simulink model "my_PMSM"  (Simulink 8.6)
settings: Solver=ode45  StartTime=0.0  StopTime=2  MaxStep=1e-5  RelTol=1e-3
model workspace (MAT data in the model file):
  Ld = 0.00019
  Lq = 0.00051
  PP = 4
  fluxM = 0.0814
values from neighbouring files (symbols this model uses):
  fluxM = 0.0814    [aaa.mat]
  Ld = 0.00019    [aaa.mat]    (also in param.m = 2e-05)
  Lq = 0.00051    [aaa.mat]    (also in param.m = 4e-05)
  PP = 4    [aaa.mat]
undefined symbols (not defined in the file or in its folder): Vdc
libraries: powerlib x6, powerlib_extras x4, simulink x1
settings Model: Creator=lenovo  LastModifiedBy=Administrator
settings OptimizationCC: InitFltsAndDblsToZero=on
settings DebuggingCC: SaveWithParameterizedLinksMsg=none  SignalResolutionControl=TryResolveAllWithWarning  MultiTaskDSMMsg=warning  MultiTaskCondExecSysMsg=none  FcnCallInpInsideContextMsg=UseLocalSettings
settings GRTTargetCC: TargetFcnLib=ansi_tfl_tmw.mat

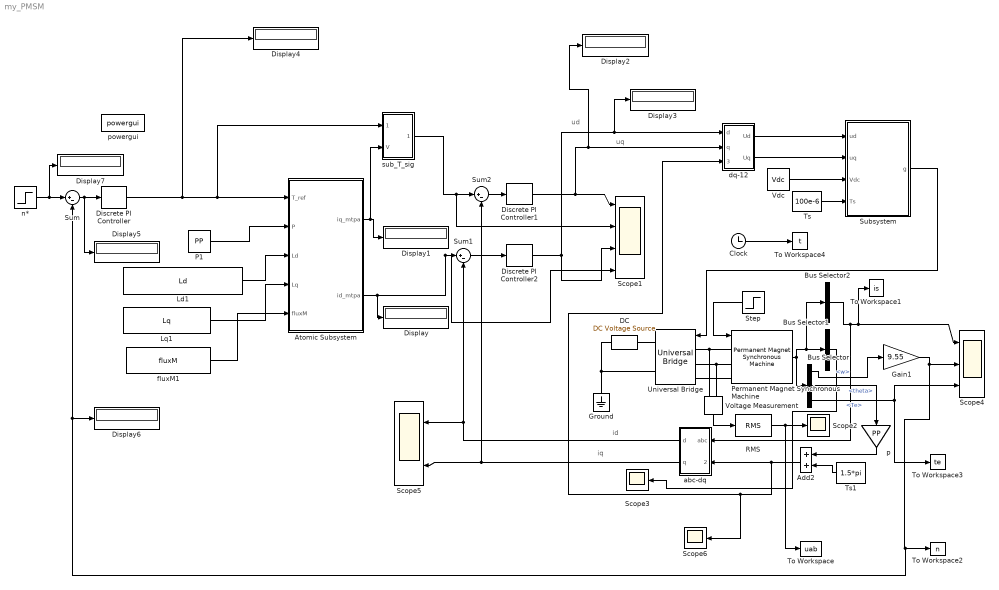
== system my_PMSM ==
  note: id
  note: iq
  note: ud
  note: uq
  Add2 : Sum
  Atomic Subsystem : Subsystem  TreatAsAtomicUnit=on
  Bus Selector : BusSelector  OutputSignals=w,theta,Te
  Bus Selector1 : BusSelector  OutputSignals=iqs,ids  OutputAsBus=on
  Bus Selector2 : BusSelector  OutputSignals=ias,ibs,ics  OutputAsBus=on
  Clock : Clock
  DC : powerlib/Electrical Sources/DC Voltage Source  Amplitude=Vdc  Measurements=None
  Discrete PI Controller : powerlib_extras/Discrete  Control Blocks/Discrete PI Controller  Kp=0.2  Ki=2  Par_Limits=[150 -150]  Init=0  Ts=100e-6
  Discrete PI Controller1 : powerlib_extras/Discrete  Control Blocks/Discrete PI Controller  Kp=1  Ki=0.015  Par_Limits=[Vdc/1.732 -1*(Vdc/1.732)]  Init=0  Ts=100e-6
  Discrete PI Controller2 : powerlib_extras/Discrete  Control Blocks/Discrete PI Controller  Kp=1  Ki=0.015  Par_Limits=[Vdc/1.732 -1*(Vdc/1.732)]  Init=0  Ts=100e-6
  Display{,1..7} (8 alike) : Display
  Gain1 : Gain  Gain=9.55
  Ground : powerlib/Elements/Ground  LConnTagsString=a
  Ld1 : Constant  Value=Ld
  "Lq1 " : Constant  Value=Lq
  P1 : Constant  Value=PP
  Permanent Magnet Synchronous Machine : powerlib/Machines/Permanent Magnet Synchronous Machine  NbPhases=3  FluxDistribution=Sinusoidal  RotorType=Salient-pole  MechanicalLoad=Torque Tm  PresetModel=No  ShowDetailedParameters=on  MeasurementBus=on  Resistance=2e-2  Inductance=8.5e-3  dqInductances=[Ld Lq]  La=0.000395  MachineConstant=Flux linkage established by magnets (V.s)  Flux=fluxM  VoltageCst=59.0573  TorqueCst=0.4884  Flat=120  Mechanical=[8e-3 0 4 0]  PolePairs=PP  InitialConditions=[0,0, 0,0]  InitialConditions5ph=[0 0 0 0 0 0]  TsPowergui=0  TsBlock=-1  RefAngle=90 degrees behind phase A axis (modified Park)
  RMS : powerlib_extras/Measurements/RMS  f1=50
  Scope1 : Scope  NumInputPorts=4
  Scope2 : Scope
  Scope3 : Scope
  Scope4 : Scope  NumInputPorts=3
  Scope5 : Scope  NumInputPorts=2
  Scope6 : Scope
  Step : Step  Time=0.8  Before=-2  After=-10  SampleTime=0
  Subsystem : Subsystem
  Sum : Sum  Inputs=|+-
  Sum1 : Sum  Inputs=|+-
  Sum2 : Sum  Inputs=|+-
  To Workspace : ToWorkspace  VariableName=uab  SampleTime=-1
  To Workspace1 : ToWorkspace  VariableName=is  SampleTime=-1
  To Workspace2 : ToWorkspace  VariableName=n  SampleTime=-1
  To Workspace3 : ToWorkspace  VariableName=te  SampleTime=-1
  To Workspace4 : ToWorkspace  VariableName=t  SampleTime=-1
  Ts : Constant  Value=100e-6
  Ts1 : Constant  Value=1.5*pi
  Universal Bridge : powerlib/Power Electronics/Universal Bridge  Arms=3  SnubberResistance=1e5  SnubberCapacitance=inf  Device=IGBT / Diodes  Ron=1e-3  Lon=0  ForwardVoltages="[  0  0  ]"  ForwardVoltage=0  GTOparameters=[ 10e-6 , 20e-6 ]  IGBTparameters=[ 1e-6 , 2e-6 ]  Measurements=None  Measurements_2=None  converterType=Rectifier
  Vdc : Constant  Value=Vdc
  Voltage Measurement : powerlib/Measurements/Voltage Measurement  PhasorSimulation=off  OutputType=Complex  PSBequivalent=0
  abc-dq : Subsystem
  dq-12 : Subsystem
  fluxM1 : Constant  Value=fluxM
  n* : Step  Time=0.4  Before=500  After=800  SampleTime=1e-5
  p : Gain  Gain=PP
  powergui : powerlib/powergui  SimulationMode=Continuous  SolverType=Tustin/Backward Euler (TBE)  SampleTime=0  frequency=60  SPID=off  DisableSnubberDevices=off  DisableRonSwitches=off  DisableVfSwitches=off  SwTol=0  DisplayEquations=off  Interpol=off  ExternalGateDelay=off  methode=off  Ts=0  FunctionMessages=off  echomessages=off  HookPort=off  EnableUseOfTLC=off  x0status=blocks  frequencyindice=0  Pbase=100e6  ErrMax=1e-4  Iterations=50  UnitsV=kV  UnitsW=MW  buscounter=0  RestoreLinks=warning  ResistiveCurrentMeasurement=off  Frange=[0:2:500]  Ylog=off  Xlog=on  ShowGrid=off  save=off  variable=ZData  structure=0  ZoomFFT=on  StartTime=0.0  cycles=1  DisplayStyle=1  fundamental=60  FreqAxis=off  MaxFrequency=1000  frequencyindicesteady=1  RmsSteady=1  display=off
  "sub_T_sig " : Subsystem
  wires:
  Sum2/1 -> Discrete PI Controller1/1
  Sum1/1 -> Discrete PI Controller2/1
  Discrete PI Controller1/1 -> Scope1/1, Display2/1, dq-12/2(q)
  Discrete PI Controller2/1 -> Display3/1, dq-12/1(d), Scope1/3
  Permanent Magnet Synchronous Machine/1 -> Bus Selector/1, Bus Selector2/1, Bus Selector1/1
  Bus Selector2/1 -> abc-dq/1(abc), Scope4/1, To Workspace1/1
  Step/1 -> Permanent Magnet Synchronous Machine/1
  Bus Selector/2 -> p/1  "<theta>"
  Bus Selector/3 -> Scope4/3, To Workspace3/1  "<Te>"
  Subsystem/1(g) -> Universal Bridge/1
  abc-dq/1(d) -> Scope5/1, Sum1/2
  abc-dq/2(q) -> Scope5/2, Sum2/2
  Gain1/1 -> Scope4/2, Display6/1, Sum/2, To Workspace2/1
  p/1 -> Add2/1
  Ts1/1 -> Add2/2
  dq-12/1(Ud) -> Subsystem/1(ud)
  dq-12/2(Uq) -> Subsystem/2(uq)
  Vdc/1 -> Subsystem/3(Vdc)
  Ts/1 -> Subsystem/4(Ts)
  RMS/1 -> Scope2/1, To Workspace/1
  Voltage Measurement/1 -> RMS/1
  Clock/1 -> To Workspace4/1
  Bus Selector/1 -> Gain1/1  "<w>"
  Atomic Subsystem/2(id_mtpa) -> Display/1, Scope1/4, Sum1/1
  P1/1 -> Atomic Subsystem/2(P)
  Ld1/1 -> Atomic Subsystem/3(Ld)
  "Lq1 "/1 -> Atomic Subsystem/4(Lq)
  fluxM1/1 -> Atomic Subsystem/5(fluxM)
  Atomic Subsystem/1(iq_mtpa) -> "sub_T_sig "/2(V), Display1/1
  "sub_T_sig "/1(Out1) -> Scope1/2, Sum2/1
  Add2/1 -> abc-dq/2(theta), Scope6/1, dq-12/3(theta)
  Sum/1 -> Display5/1, Discrete PI Controller/1
  n*/1 -> Display7/1, Sum/1
  Discrete PI Controller/1 -> Display4/1, "sub_T_sig "/1(Sig), Atomic Subsystem/1(T_ref)
  Bus Selector1/1 -> Scope3/1
  connections:
  Universal Bridge/LConn1 -- Permanent Magnet Synchronous Machine/LConn1 -- Voltage Measurement/LConn1
  Universal Bridge/LConn2 -- Permanent Magnet Synchronous Machine/LConn2 -- Voltage Measurement/LConn2
  Universal Bridge/LConn3 -- Permanent Magnet Synchronous Machine/LConn3
  DC/LConn1 -- Universal Bridge/RConn2 -- Ground/LConn1
  DC/RConn1 -- Universal Bridge/RConn1

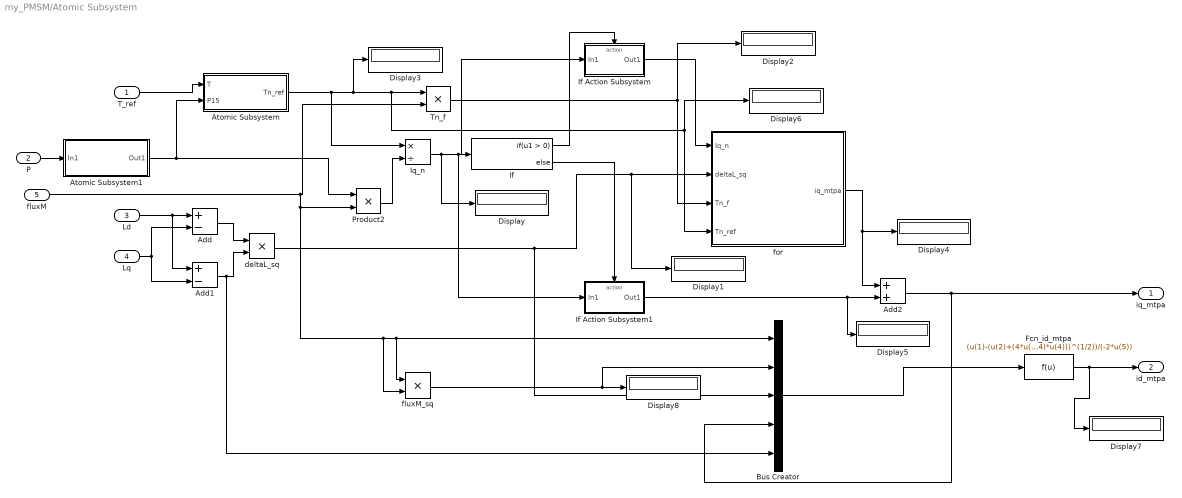
== system my_PMSM/Atomic Subsystem ==
  T_ref : Inport
  P : Inport  Port=2
  Ld : Inport  Port=3
  Lq : Inport  Port=4
  fluxM : Inport  Port=5
  Add : Sum  Inputs=+-
  Add1 : Sum  Inputs=+-
  Add2 : Sum
  Atomic Subsystem : Subsystem  TreatAsAtomicUnit=on
  Atomic Subsystem1 : Subsystem  TreatAsAtomicUnit=on
  Bus Creator : BusCreator  Inputs=5
  Display{,1..8} (9 alike) : Display
  Fcn_id_mtpa : Fcn  Expr=(u(1)-(u(2)+(4*u(3)*u(4)*u(4)))^(1/2))/(-2*u(5))
  If : If
  If Action Subsystem : Subsystem  TreatAsAtomicUnit=on
  If Action Subsystem1 : Subsystem  TreatAsAtomicUnit=on
  Iq_n : Product  Inputs=*/
  Product2 : Product
  Tn_f : Product
  deltaL_sq : Product
  fluxM_sq : Product
  "for " : Subsystem  TreatAsAtomicUnit=on
  iq_mtpa : Outport
  id_mtpa : Outport  Port=2
  wires:
  T_ref/1 -> Atomic Subsystem/1(T)
  P/1 -> Atomic Subsystem1/1(In1)
  Atomic Subsystem1/1(Out1) -> Product2/1, Atomic Subsystem/2(P15)
  Ld/1 -> Add1/1, Add/1
  Lq/1 -> Add/2, Add1/2
  Add/1 -> deltaL_sq/1
  Add1/1 -> Bus Creator/5, deltaL_sq/2
  Atomic Subsystem/1(Tn_ref) -> Iq_n/1, Display3/1, Display6/1, "for "/4(Tn_ref), Tn_f/1
  fluxM/1 -> fluxM_sq/2, fluxM_sq/1, Bus Creator/1, Product2/2, Tn_f/2
  Product2/1 -> Iq_n/2
  Iq_n/1 -> Display/1, If Action Subsystem1/1(In1), If Action Subsystem/1(In1), If/1
  deltaL_sq/1 -> Bus Creator/3, Display1/1, "for "/2(deltaL_sq)
  Tn_f/1 -> "for "/3(Tn_f), Display2/1
  If/1 -> If Action Subsystem/Action
  If Action Subsystem/1(Out1) -> "for "/1("Iq_n ")
  If/2 -> If Action Subsystem1/Action
  Add2/1 -> Bus Creator/4, iq_mtpa/1
  If Action Subsystem1/1(Out1) -> Display5/1, Add2/2
  "for "/1(iq_mtpa) -> Display4/1, Add2/1
  Fcn_id_mtpa/1 -> Display7/1, id_mtpa/1
  Bus Creator/1 -> Fcn_id_mtpa/1
  fluxM_sq/1 -> Display8/1, Bus Creator/2

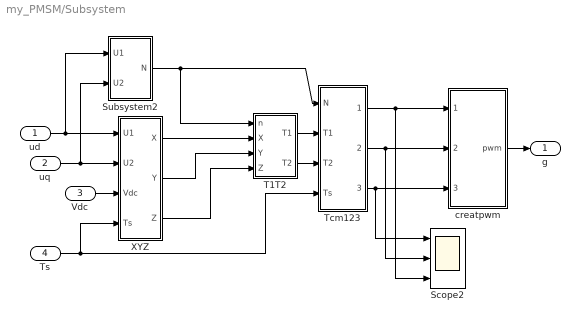
== system my_PMSM/Subsystem ==
  ud : Inport
  uq : Inport  Port=2
  Vdc : Inport  Port=3
  Ts : Inport  Port=4
  Scope2 : Scope  NumInputPorts=3
  Subsystem2 : Subsystem
  T1T2 : Subsystem
  Tcm123 : Subsystem
  XYZ : Subsystem
  creatpwm : Subsystem
  g : Outport
  wires:
  Subsystem2/1(N) -> Tcm123/1(N), T1T2/1(n)
  XYZ/1(X) -> T1T2/2(X)
  XYZ/2(Y) -> T1T2/3(Y)
  XYZ/3(Z) -> T1T2/4(Z)
  T1T2/1(T1) -> Tcm123/2(T1)
  T1T2/2(T2) -> Tcm123/3(T2)
  Tcm123/1(Tcm1) -> creatpwm/1(Tcm1), Scope2/3
  Tcm123/2(Tcm2) -> creatpwm/2(Tcm2), Scope2/2
  Tcm123/3(Tcm3) -> creatpwm/3(Tcm3), Scope2/1
  ud/1 -> Subsystem2/1(U1), XYZ/1(U1)
  uq/1 -> Subsystem2/2(U2), XYZ/2(U2)
  Ts/1 -> Tcm123/4(Ts), XYZ/4(Ts)
  creatpwm/1(pwm) -> g/1
  Vdc/1 -> XYZ/3(Vdc)

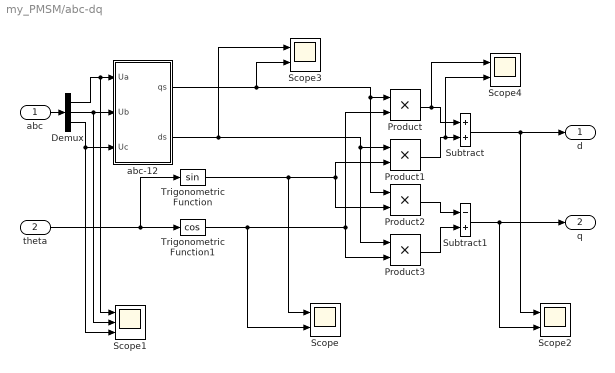
== system my_PMSM/abc-dq ==
  abc : Inport
  theta : Inport  Port=2
  Demux : Demux  Outputs=3
  Product{,1..3} (4 alike) : Product  RndMeth=Zero
  Scope{,2..4} (4 alike) : Scope  NumInputPorts=2
  Scope1 : Scope  NumInputPorts=3
  Subtract : Sum
  Subtract1 : Sum  Inputs=-+
  Trigonometric Function : Trigonometry
  Trigonometric Function1 : Trigonometry  Operator=cos
  abc-12 : Subsystem
  d : Outport
  q : Outport  Port=2
  wires:
  Demux/3 -> Scope1/3, abc-12/3(Uc)
  Demux/2 -> Scope1/2, abc-12/2(Ub)
  Demux/1 -> Scope1/1, abc-12/1(Ua)
  abc/1 -> Demux/1
  abc-12/2(ds) -> Scope3/1, Product3/1, Product1/1
  abc-12/1(qs) -> Scope3/2, Product2/1, Product/1
  Subtract1/1 -> Scope2/2, q/1
  Subtract/1 -> Scope2/1, d/1
  Product3/1 -> Subtract1/2
  Product2/1 -> Subtract1/1
  Product1/1 -> Scope4/2, Subtract/2
  Product/1 -> Scope4/1, Subtract/1
  theta/1 -> Trigonometric Function1/1, Trigonometric Function/1
  Trigonometric Function1/1 -> Scope/2, Product3/2, Product/2
  Trigonometric Function/1 -> Scope/1, Product2/2, Product1/2

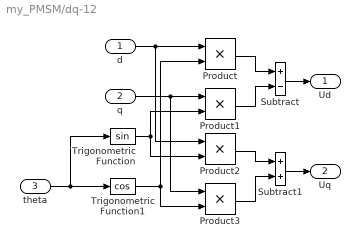
== system my_PMSM/dq-12 ==
  d : Inport
  q : Inport  Port=2
  theta : Inport  Port=3
  Product{,1..3} (4 alike) : Product  RndMeth=Zero
  Subtract : Sum  Inputs=+-
  Subtract1 : Sum
  Trigonometric Function : Trigonometry
  Trigonometric Function1 : Trigonometry  Operator=cos
  Ud : Outport
  Uq : Outport  Port=2
  wires:
  Subtract1/1 -> Uq/1
  Subtract/1 -> Ud/1
  Product3/1 -> Subtract1/2
  Product2/1 -> Subtract1/1
  Product1/1 -> Subtract/2
  Product/1 -> Subtract/1
  theta/1 -> Trigonometric Function/1, Trigonometric Function1/1
  q/1 -> Product3/1, Product1/1
  d/1 -> Product2/1, Product/1
  Trigonometric Function1/1 -> Product3/2, Product/2
  Trigonometric Function/1 -> Product2/2, Product1/2

== system my_PMSM/sub_T_sig  ==
  Sig : Inport
  V : Inport  Port=2
  Add1 : Sum
  Gain : Gain  Gain=-1
  If : If  IfExpression=u1 < 0
  If 1 : Subsystem  TreatAsAtomicUnit=on
  If 2 : Subsystem  TreatAsAtomicUnit=on
  Out1 : Outport
  wires:
  If 1/1(Out1) -> Add1/2
  If/2 -> If 1/Action
  Gain/1 -> Add1/1
  If/1 -> If 2/Action
  If 2/1(Out1) -> Gain/1
  Add1/1 -> Out1/1
  V/1 -> If 2/1(In1), If 1/1(In1)
  Sig/1 -> If/1

== system my_PMSM/Atomic Subsystem/Atomic Subsystem ==
  T : Inport
  P15 : Inport  Port=2
  Abs : Abs
  Divide : Product  Inputs=*/
  Tn_ref : Outport
  wires:
  T/1 -> Abs/1
  Abs/1 -> Divide/1
  P15/1 -> Divide/2
  Divide/1 -> Tn_ref/1

== system my_PMSM/Atomic Subsystem/Atomic Subsystem1 ==
  In1 : Inport
  Gain : Gain  Gain=1.5
  Out1 : Outport
  wires:
  In1/1 -> Gain/1
  Gain/1 -> Out1/1

== system my_PMSM/Atomic Subsystem/If Action Subsystem ==
  In1 : Inport
  Action Port : ActionPort  ActionType=then
  Out1 : Outport
  wires:
  In1/1 -> Out1/1

== system my_PMSM/Atomic Subsystem/If Action Subsystem1 ==
  In1 : Inport
  Action Port : ActionPort  ActionType=else
  Out1 : Outport
  wires:
  In1/1 -> Out1/1

== system my_PMSM/Atomic Subsystem/for  ==
  "Iq_n " : Inport
  deltaL_sq : Inport  Port=2
  Tn_f : Inport  Port=3
  Tn_ref : Inport  Port=4
  Display1 : Display
  Display2 : Display
  Display4 : Display
  "for1 " : Subsystem  TreatAsAtomicUnit=on
  for1 1 : Subsystem  TreatAsAtomicUnit=on
  for1 2 : Subsystem  TreatAsAtomicUnit=on
  iq_mtpa : Outport
  wires:
  "Iq_n "/1 -> "for1 "/1("Iq_n ")
  "for1 "/1(iq_mtpa) -> Display2/1, for1 1/1("Iq_n ")
  for1 1/1(iq_mtpa) -> Display4/1, for1 2/1("Iq_n ")
  deltaL_sq/1 -> for1 2/2(deltaL_sq), for1 1/2(deltaL_sq), "for1 "/2(deltaL_sq)
  Tn_f/1 -> for1 2/3(Tn_f), for1 1/3(Tn_f), "for1 "/3(Tn_f)
  Tn_ref/1 -> for1 2/4(Tn_ref), for1 1/4(Tn_ref), "for1 "/4(Tn_ref)
  for1 2/1(iq_mtpa) -> Display1/1, iq_mtpa/1

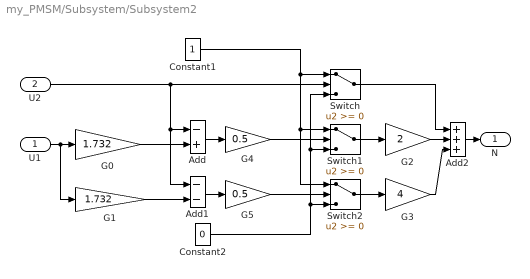
== system my_PMSM/Subsystem/Subsystem2 ==
  U1 : Inport
  U2 : Inport  Port=2
  Add : Sum  Inputs=-+
  Add1 : Sum  Inputs=--
  Add2 : Sum  Inputs=+++
  Constant1 : Constant
  Constant2 : Constant  Value=0
  G0 : Gain  Gain=1.732
  G1 : Gain  Gain=1.732
  G2 : Gain  Gain=2
  G3 : Gain  Gain=4
  G4 : Gain  Gain=0.5
  G5 : Gain  Gain=0.5
  Switch : Switch
  Switch1 : Switch
  Switch2 : Switch
  N : Outport
  wires:
  Add2/1 -> N/1
  Switch/1 -> Add2/1
  G3/1 -> Add2/3
  G2/1 -> Add2/2
  Switch1/1 -> G2/1
  Switch2/1 -> G3/1
  Add1/1 -> G5/1
  Constant2/1 -> Switch2/3, Switch1/3, Switch/3
  Add/1 -> G4/1
  Constant1/1 -> Switch2/1, Switch1/1, Switch/1
  U2/1 -> Add1/1, Add/1, Switch/2
  G1/1 -> Add1/2
  U1/1 -> G1/1, G0/1
  G0/1 -> Add/2
  G4/1 -> Switch1/2
  G5/1 -> Switch2/2

== system my_PMSM/Subsystem/T1T2 ==
  n : Inport
  X : Inport  Port=2
  Y : Inport  Port=3
  Z : Inport  Port=4
  G1 : Gain  Gain=-1
  G2 : Gain  Gain=-1
  G3 : Gain  Gain=-1
  Multiport Switch : MultiPortSwitch  Inputs=6
  Multiport Switch1 : MultiPortSwitch  Inputs=6
  T1 : Outport
  T2 : Outport  Port=2
  wires:
  G2/1 -> Multiport Switch1/6, Multiport Switch/7
  G3/1 -> Multiport Switch1/7, Multiport Switch/4
  G1/1 -> Multiport Switch1/3, Multiport Switch/5
  Z/1 -> Multiport Switch1/5, Multiport Switch/2, G3/1
  Y/1 -> Multiport Switch1/2, Multiport Switch/3, G2/1
  X/1 -> Multiport Switch1/4, Multiport Switch/6, G1/1
  n/1 -> Multiport Switch1/1, Multiport Switch/1
  Multiport Switch1/1 -> T2/1
  Multiport Switch/1 -> T1/1

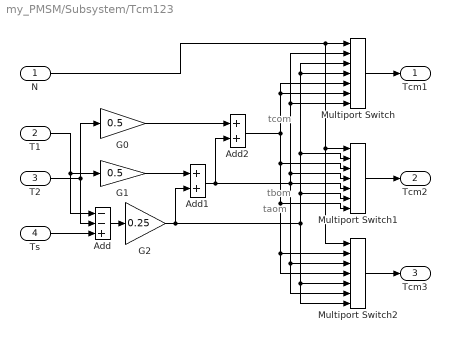
== system my_PMSM/Subsystem/Tcm123 ==
  note: taom
  note: tbom
  note: tcom
  N : Inport
  T1 : Inport  Port=2
  T2 : Inport  Port=3
  Ts : Inport  Port=4
  Add : Sum  Inputs=--+
  Add1 : Sum
  Add2 : Sum
  G0 : Gain  Gain=0.5
  G1 : Gain  Gain=0.5
  G2 : Gain  Gain=0.25
  Multiport Switch : MultiPortSwitch  Inputs=6
  Multiport Switch1 : MultiPortSwitch  Inputs=6
  Multiport Switch2 : MultiPortSwitch  Inputs=6
  Tcm1 : Outport
  Tcm2 : Outport  Port=2
  Tcm3 : Outport  Port=3
  wires:
  Add2/1 -> Multiport Switch1/3, Multiport Switch2/4, Multiport Switch2/2, Multiport Switch1/7, Multiport Switch/5, Multiport Switch/6
  Add1/1 -> Multiport Switch2/6, Multiport Switch2/3, Multiport Switch1/5, Multiport Switch1/4, Multiport Switch/2, Multiport Switch/7, Add2/2
  G2/1 -> Multiport Switch2/5, Multiport Switch2/7, Multiport Switch1/6, Multiport Switch1/2, Multiport Switch/4, Multiport Switch/3, Add1/2
  G1/1 -> Add1/1
  G0/1 -> Add2/1
  Add/1 -> G2/1
  Ts/1 -> Add/3
  T2/1 -> Add/2, G0/1
  T1/1 -> Add/1, G1/1
  Multiport Switch2/1 -> Tcm3/1
  Multiport Switch1/1 -> Tcm2/1
  N/1 -> Multiport Switch/1, Multiport Switch2/1, Multiport Switch1/1
  Multiport Switch/1 -> Tcm1/1

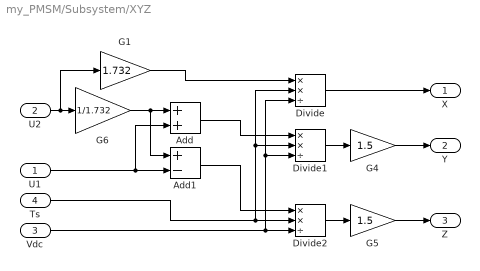
== system my_PMSM/Subsystem/XYZ ==
  U1 : Inport
  U2 : Inport  Port=2
  Vdc : Inport  Port=3
  Ts : Inport  Port=4
  Add : Sum
  Add1 : Sum  Inputs=+-
  Divide : Product  Inputs=**/
  Divide1 : Product  Inputs=**/
  Divide2 : Product  Inputs=**/
  G1 : Gain  Gain=1.732
  G4 : Gain  Gain=1.5
  G5 : Gain  Gain=1.5
  G6 : Gain  Gain=1/1.732
  X : Outport
  Y : Outport  Port=2
  Z : Outport  Port=3
  wires:
  Divide/1 -> X/1
  G4/1 -> Y/1
  G5/1 -> Z/1
  Divide2/1 -> G5/1
  Divide1/1 -> G4/1
  Vdc/1 -> Divide/3, Divide1/3, Divide2/3
  Ts/1 -> Divide/2, Divide1/2, Divide2/2
  Add1/1 -> Divide2/1
  Add/1 -> Divide1/1
  G1/1 -> Divide/1
  U1/1 -> Add1/2, Add/2
  U2/1 -> G1/1, G6/1
  G6/1 -> Add/1, Add1/1

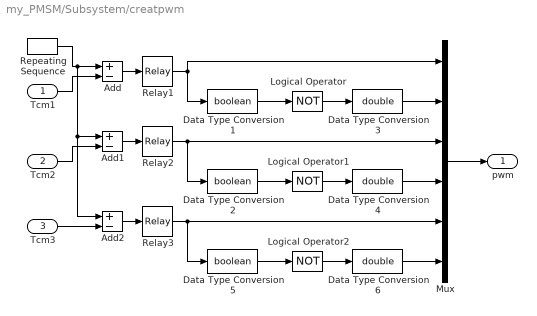
== system my_PMSM/Subsystem/creatpwm ==
  Tcm1 : Inport
  Tcm2 : Inport  Port=2
  Tcm3 : Inport  Port=3
  Add : Sum  Inputs=+-
  Add1 : Sum  Inputs=+-
  Add2 : Sum  Inputs=+-
  Data Type Conversion1 : DataTypeConversion  OutDataTypeStr=boolean
  Data Type Conversion2 : DataTypeConversion  OutDataTypeStr=boolean
  Data Type Conversion3 : DataTypeConversion  OutDataTypeStr=double
  Data Type Conversion4 : DataTypeConversion  OutDataTypeStr=double
  Data Type Conversion5 : DataTypeConversion  OutDataTypeStr=boolean
  Data Type Conversion6 : DataTypeConversion  OutDataTypeStr=double
  Logical Operator : Logic  Operator=NOT  AllPortsSameDT=off  OutDataTypeStr=boolean
  Logical Operator1 : Logic  Operator=NOT  AllPortsSameDT=off  OutDataTypeStr=boolean
  Logical Operator2 : Logic  Operator=NOT  AllPortsSameDT=off  OutDataTypeStr=boolean
  Mux : Mux  Inputs=6
  Relay1 : Relay
  Relay2 : Relay
  Relay3 : Relay
  Repeating Sequence : simulink/Sources/Repeating Sequence  rep_seq_t=[0 5e-4]  rep_seq_y=[-0.05 0.05]
  pwm : Outport
  wires:
  Mux/1 -> pwm/1
  Tcm1/1 -> Add/2
  Logical Operator2/1 -> Data Type Conversion6/1
  Data Type Conversion5/1 -> Logical Operator2/1
  Logical Operator1/1 -> Data Type Conversion4/1
  Data Type Conversion2/1 -> Logical Operator1/1
  Logical Operator/1 -> Data Type Conversion3/1
  Data Type Conversion1/1 -> Logical Operator/1
  Relay1/1 -> Mux/1, Data Type Conversion1/1
  Relay3/1 -> Mux/5, Data Type Conversion5/1
  Relay2/1 -> Mux/3, Data Type Conversion2/1
  Add2/1 -> Relay3/1
  Add1/1 -> Relay2/1
  Add/1 -> Relay1/1
  Tcm3/1 -> Add2/2
  Tcm2/1 -> Add1/2
  Data Type Conversion3/1 -> Mux/2
  Data Type Conversion4/1 -> Mux/4
  Data Type Conversion6/1 -> Mux/6
  Repeating Sequence/1 -> Add/1, Add1/1, Add2/1

== system my_PMSM/abc-dq/abc-12 ==
  Ua : Inport
  Ub : Inport  Port=2
  Uc : Inport  Port=3
  Add1 : Sum  Inputs=+-
  G2 : Gain  Gain=1/1.732
  qs : Outport
  ds : Outport  Port=2
  wires:
  Ua/1 -> qs/1
  Ub/1 -> Add1/1
  Uc/1 -> Add1/2
  Add1/1 -> G2/1
  G2/1 -> ds/1

== system my_PMSM/sub_T_sig /If 1 ==
  In1 : Inport
  Action Port : ActionPort  ActionType=else
  Out1 : Outport
  wires:
  In1/1 -> Out1/1

== system my_PMSM/sub_T_sig /If 2 ==
  In1 : Inport
  Action Port : ActionPort  ActionType=then
  Out1 : Outport
  wires:
  In1/1 -> Out1/1

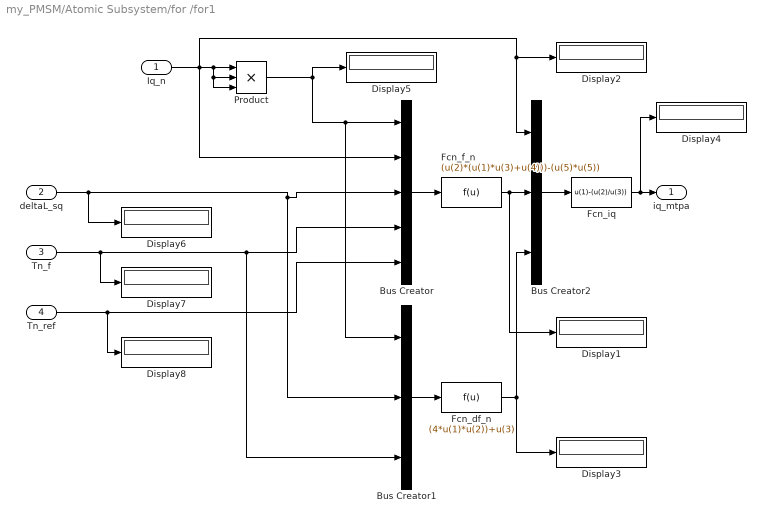
== system my_PMSM/Atomic Subsystem/for /for1  ==
  "Iq_n " : Inport
  deltaL_sq : Inport  Port=2
  Tn_f : Inport  Port=3
  Tn_ref : Inport  Port=4
  Bus Creator : BusCreator  Inputs=5
  Bus Creator1 : BusCreator  Inputs=3
  Bus Creator2 : BusCreator  Inputs=3
  Display{1..8} (8 alike) : Display
  Fcn_df_n : Fcn  Expr=(4*u(1)*u(2))+u(3)
  Fcn_f_n : Fcn  Expr=(u(2)*(u(1)*u(3)+u(4)))-(u(5)*u(5))
  Fcn_iq : Fcn  Expr=u(1)-(u(2)/u(3))
  Product : Product  Inputs=3
  iq_mtpa : Outport
  wires:
  "Iq_n "/1 -> Product/3, Product/2, Product/1, Bus Creator2/1, Display2/1, Bus Creator/2
  Bus Creator/1 -> Fcn_f_n/1
  Product/1 -> Display5/1, Bus Creator1/1, Bus Creator/1
  deltaL_sq/1 -> Display6/1, Bus Creator1/2, Bus Creator/3
  Tn_f/1 -> Display7/1, Bus Creator1/3, Bus Creator/4
  Tn_ref/1 -> Display8/1, Bus Creator/5
  Bus Creator1/1 -> Fcn_df_n/1
  Fcn_f_n/1 -> Display1/1, Bus Creator2/2
  Fcn_df_n/1 -> Display3/1, Bus Creator2/3
  Bus Creator2/1 -> Fcn_iq/1
  Fcn_iq/1 -> Display4/1, iq_mtpa/1

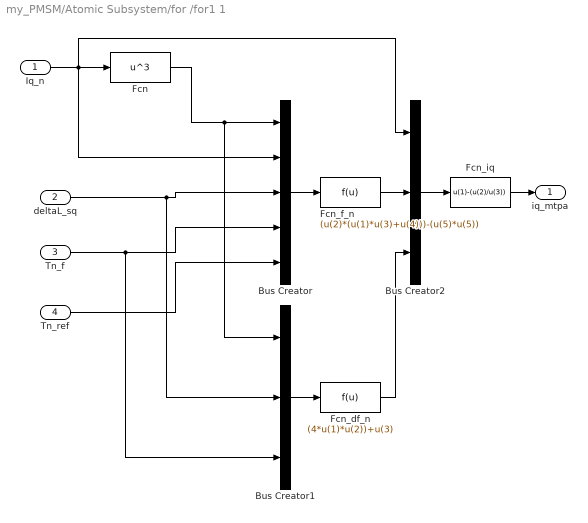
== system my_PMSM/Atomic Subsystem/for /for1 1 ==
  "Iq_n " : Inport
  deltaL_sq : Inport  Port=2
  Tn_f : Inport  Port=3
  Tn_ref : Inport  Port=4
  Bus Creator : BusCreator  Inputs=5
  Bus Creator1 : BusCreator  Inputs=3
  Bus Creator2 : BusCreator  Inputs=3
  Fcn : Fcn  Expr=u^3
  Fcn_df_n : Fcn  Expr=(4*u(1)*u(2))+u(3)
  Fcn_f_n : Fcn  Expr=(u(2)*(u(1)*u(3)+u(4)))-(u(5)*u(5))
  Fcn_iq : Fcn  Expr=u(1)-(u(2)/u(3))
  iq_mtpa : Outport
  wires:
  "Iq_n "/1 -> Bus Creator2/1, Bus Creator/2, Fcn/1
  Bus Creator/1 -> Fcn_f_n/1
  Fcn/1 -> Bus Creator1/1, Bus Creator/1
  deltaL_sq/1 -> Bus Creator1/2, Bus Creator/3
  Tn_f/1 -> Bus Creator1/3, Bus Creator/4
  Tn_ref/1 -> Bus Creator/5
  Bus Creator1/1 -> Fcn_df_n/1
  Fcn_f_n/1 -> Bus Creator2/2
  Fcn_df_n/1 -> Bus Creator2/3
  Bus Creator2/1 -> Fcn_iq/1
  Fcn_iq/1 -> iq_mtpa/1

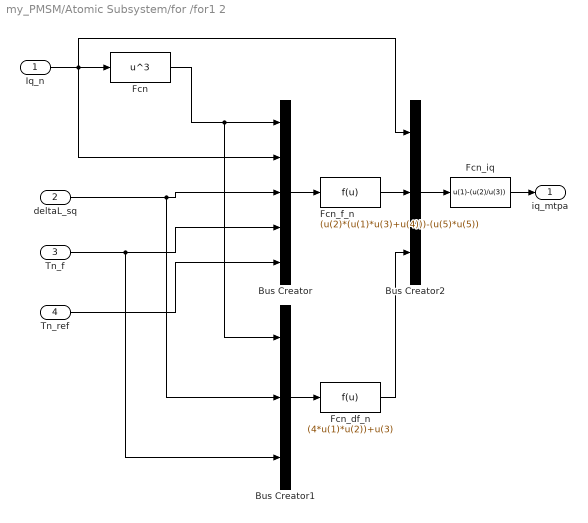
== system my_PMSM/Atomic Subsystem/for /for1 2 ==
  "Iq_n " : Inport
  deltaL_sq : Inport  Port=2
  Tn_f : Inport  Port=3
  Tn_ref : Inport  Port=4
  Bus Creator : BusCreator  Inputs=5
  Bus Creator1 : BusCreator  Inputs=3
  Bus Creator2 : BusCreator  Inputs=3
  Fcn : Fcn  Expr=u^3
  Fcn_df_n : Fcn  Expr=(4*u(1)*u(2))+u(3)
  Fcn_f_n : Fcn  Expr=(u(2)*(u(1)*u(3)+u(4)))-(u(5)*u(5))
  Fcn_iq : Fcn  Expr=u(1)-(u(2)/u(3))
  iq_mtpa : Outport
  wires:
  "Iq_n "/1 -> Bus Creator2/1, Bus Creator/2, Fcn/1
  Bus Creator/1 -> Fcn_f_n/1
  Fcn/1 -> Bus Creator1/1, Bus Creator/1
  deltaL_sq/1 -> Bus Creator1/2, Bus Creator/3
  Tn_f/1 -> Bus Creator1/3, Bus Creator/4
  Tn_ref/1 -> Bus Creator/5
  Bus Creator1/1 -> Fcn_df_n/1
  Fcn_f_n/1 -> Bus Creator2/2
  Fcn_df_n/1 -> Bus Creator2/3
  Bus Creator2/1 -> Fcn_iq/1
  Fcn_iq/1 -> iq_mtpa/1
